simulink model "Capture"  (Simulink 7.0)
settings: Solver=ode1  StartTime=0.0  StopTime=10  FixedStep=0.001  RelTol=1e-3
undefined symbols (not defined in the file or in its folder): Model_626, Sensoray
libraries: rtwinlib x2
settings Model: Creator=user  LastModifiedBy=user  SimulationMode=external  ExtModeTrigDuration=15100  BufferReuse=off
settings SolverCC: PositivePriorityOrder=on
settings OptimizationCC: BooleanDataType=off  InlineInvariantSignals=on  OptimizeBlockIOStorage=off  BufferReuse=off  ExpressionFolding=off  LocalBlockOutputs=off
settings RTWCC: SystemTargetFile=rtwin.tlc  TemplateMakefile=rtwin.tmf  Description=Real-Time Windows Target  ProcessScript=rtwin_make_rtw_hook
settings RTWinTargetCC: GenFloatMathFcnCalls=ANSI_C  ModelReferenceCompliant=off  CompOptLevelCompliant=off  PortableWordSizes=off  CCOptimize=on

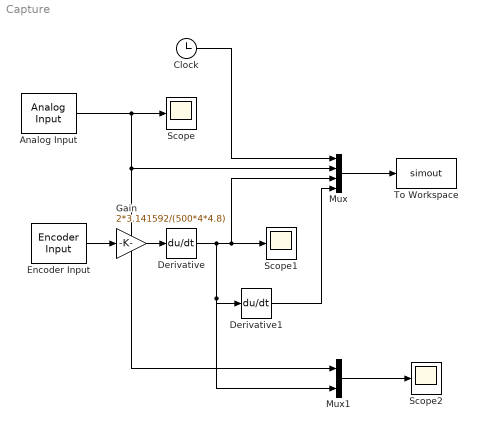
== system Capture ==
  Analog Input : rtwinlib/Analog Input  SampleTime=-1  DrvName=Sensoray/Model_626  DrvAddress=4294967295  DrvOptions=zeros(1,0)  Channels=1  RangeMode=1  VoltRange=1  DataType=1
      settings: AttributesFormatString=Sensoray\nModel 626 [auto]
  Clock : Clock
      settings: Decimation=10
  Derivative : Derivative
  Derivative1 : Derivative
  Encoder Input : rtwinlib/Encoder Input  SampleTime=-1  DrvName=Sensoray/Model_626  DrvAddress=4294967295  DrvOptions=zeros(1,0)  Channels=[4]  QuadMode=3  IndexPulse=2  InputFilter=Inf  DataType=1
      settings: AttributesFormatString=Sensoray\nModel 626 [auto]
  Gain : Gain  Gain=2*3.141592/(500*4*4.8)  ParameterDataType=sfix(16)  ParameterScaling=2^0  OutDataType=sfix(16)  OutScaling=2^0
  Mux : Mux
  Mux1 : Mux  Inputs=2
  Scope : Scope
      settings: TimeRange=10  YMin=-3  YMax=10
  Scope1 : Scope
      settings: TimeRange=10  YMin=-11  YMax=100
  Scope2 : Scope
      settings: TimeRange=10  YMin=-11  YMax=100  SaveName=ScopeData2
  To Workspace : ToWorkspace  VariableName=simout  SampleTime=-1  SaveFormat=Structure
  wires:
  Encoder Input/1 -> Gain/1
  Analog Input/1 -> Scope/1, Mux/2, Mux1/1
  Gain/1 -> Derivative/1
  Derivative/1 -> Scope1/1, Mux/3, Derivative1/1, Mux1/2
  Clock/1 -> Mux/1
  Mux/1 -> To Workspace/1
  Derivative1/1 -> Mux/4
  Mux1/1 -> Scope2/1
